simulink model "task9_2"  (R2017a)
settings: Solver=VariableStepAuto  StartTime=0.0  StopTime=10.0  RelTol=1e-3
values from neighbouring files (symbols this model uses):
  A = [0 1 0 0; -k_s/m_s -c_s/m_s k_s/m_s c_s/m_s; 0 0 0 1; k_s/m_p c_s/m_p -(k_s+k_p)/m_p -(c_s+c_p)/m_p]    [task6.3.m]    (also in task64.m = [0 1 0 0; -k_s/m_s -T/m_s k_s/m_s 0; 0 0 0 1; k_s/m_p T/m_p ; task82.m = [0 1 0 0;(-k1-k2)/m (-c1-c2)/m (k1*l1-k2*l2)/m (l1*c1-l2*c2); task92.m = [0 1 0 0;(-k1-k2)/m -cz/m (k1*l1-k2*l2)/m 0;0 0 0 1;(k1*l1-k; task9_2mod.m = [0 1 0 0)
  B = [0 0; 0 0; 0 0; c_p/m_p k_p/m_p]    [task6.3.m]    (also in task64.m = [0 0; 0 0; 0 0; k_p/m_p c_p/m_p]; task82.m = [0 0 0 0;k1/m c1/m k2/m c2/m;0 0 0 0;-k1*l1/j -c1*l1/j k2*l2; task92.m = [0 0;k1/m k2/m;0 0;-k1*l1/j -k2*l2/j]; task9_2mod.m = [0 0 0 0)
  C = [1 0 0 0]    [task6.3.m]    (also in task64.m = [1 0 0 0;0 0 0 0 ;0 0 0 0;0 0 0 0;]; task82.m = [1 0 0 0;0 0 0 0;0 0 1 0;0 0 0 0]; task92.m = [0 1 0 0;0 0 0 1]; task9_2mod.m = [1 0 0 0;0 1 0 0;0 0 1 0;0 0 0 1])
  D = 0    [task6.3.m]    (also in task64.m = [0 0;0 0;0 0;0 0]; task82.m = [0 0 0 0;0 0 0 0;0 0 0 0;0 0 0 0]; task92.m = [0 0 0 0;0 0 0 0;0 0 0 0;0 0 0 0]; task9_2mod.m = [0 0 0 0;0 0 0 0;0 0 0 0;0 0 0 0])
undefined symbols (not defined in the file or in its folder): sigbuilder_block
settings Model: Creator=utsav  LastModifiedBy=mitoa

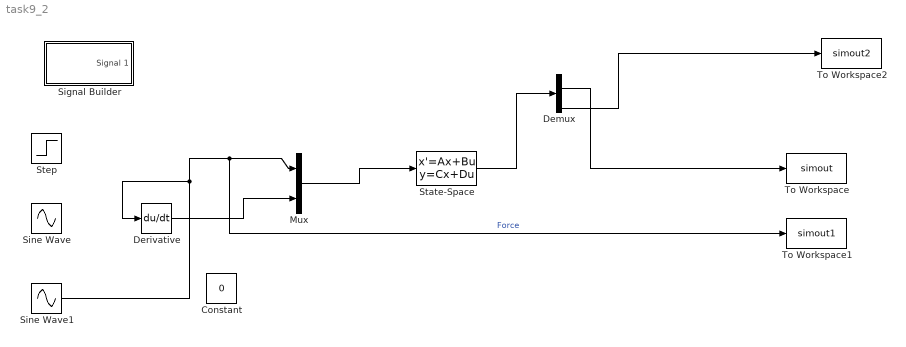
== system task9_2 ==
  Constant : Constant  Value=0
  Demux : Demux
  Derivative : Derivative
  Mux : Mux  Inputs=2
  Signal Builder : Subsystem  Tag=STV Subsys  LoadFcn=sigbuilder_block('load');  StartFcn=sigbuilder_block('start');  StopFcn=sigbuilder_block('stop');  ClipboardFcn=sigbuilder_block('clipboard');  mask(Sigbuilder block){tuvar=[0:10]}
      mask help: Simulink:masks:SigbuilderBlock_MD
      mask init:
      | if ~strcmp(get_param(bdroot(gcbh),'SimulationStatus'),'stopped') tuvar = sigbuilder_block('maskInit'); end
      settings: CopyFcn=sigbuilder_block('copy');  DeleteFcn=sigbuilder_block('delete');  ModelCloseFcn=sigbuilder_block('modelClose');  PreSaveFcn=sigbuilder_block('preSave');  PauseFcn=sigbuilder_block('pause');  ContinueFcn=sigbuilder_block('continue');  NameChangeFcn=sigbuilder_block('namechange');  OpenFcn=sigbuilder_block('open',[437.6 199.2 550.4 400 ]);  CloseFcn=sigbuilder_block('close');
      mask Display: plot(0, 0, 100, 100,[2, 2, 32, 32, 2], [68, 8, 8, 68, 68],[32, 2], [38, 38], [32, 19, 2],[53, 60, 44], [32, 17, 17, 2],[16, 16, 31, 31]);txt = getActiveGroup(gcbh);text(2, 100, txt,'verticalAlignment', 'top');
  Sine Wave : Sin  Amplitude=0.01  Frequency=6.282  SampleTime=0
  Sine Wave1 : Sin  Amplitude=0.01  Frequency=50.256  SampleTime=0
  State-Space : StateSpace  A=A  B=B  C=C  D=D  X0=0
  Step : Step  After=0.05  SampleTime=0
  To Workspace : ToWorkspace  VariableName=simout  SaveFormat=Timeseries  SampleTime=-1
  To Workspace1 : ToWorkspace  VariableName=simout1  SaveFormat=Timeseries  SampleTime=-1
  To Workspace2 : ToWorkspace  VariableName=simout2  SaveFormat=Timeseries  SampleTime=-1
  wires:
  Sine Wave1/1 -> To Workspace1/1, Mux/1, Derivative/1  "Force"
  Mux/1 -> State-Space/1
  Derivative/1 -> Mux/2
  State-Space/1 -> Demux/1
  Demux/2 -> To Workspace/1
  Demux/4 -> To Workspace2/1

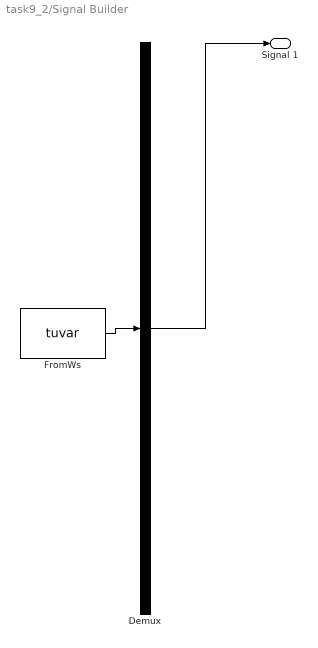
== system task9_2/Signal Builder ==
  Demux : Demux  Tag=STV Demux  Outputs=1
  FromWs : FromWorkspace  Tag=STV FromWs  VariableName=tuvar  SampleTime=0
      SigBuilderData=|
      | common.afterFinalStr = 'Extrapolate'
      | common.sampleTime = 0
      | dataSet.timeRange = [0 10]
      | dataSet.name = 'Group 1'
      | sbobj.Groups.Name = 'Group 1'
      | sbobj.Groups.Signals.Name = 'Signal 1'
      | sbobj.Groups.Signals.XData = [0 1 1 10]
      | sbobj.Groups.Signals.YData = [0.03 0.03 0 0]
  Signal 1 : Outport  Tag=STV Outport
  wires:
  Demux/1 -> Signal 1/1
  FromWs/1 -> Demux/1
